simulink model "system_simulation"  (R2024a)
settings: Solver=VariableStepAuto  StartTime=0.0  StopTime=1  RelTol=1e-3
undefined symbols (not defined in the file or in its folder): A, B, C, F, FI
settings Model: Creator=balder  LastModifiedBy=balder

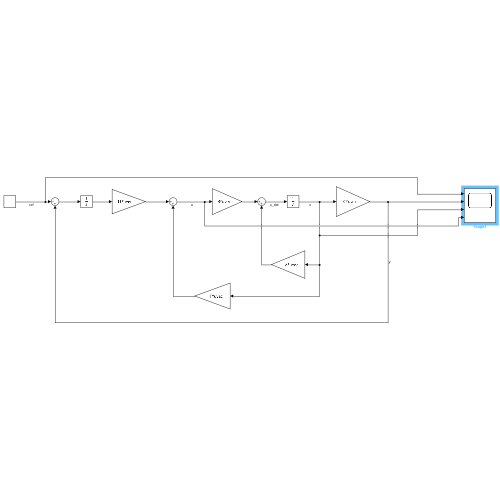
[thumbnail: Simulink's stored preview of the top-level diagram]
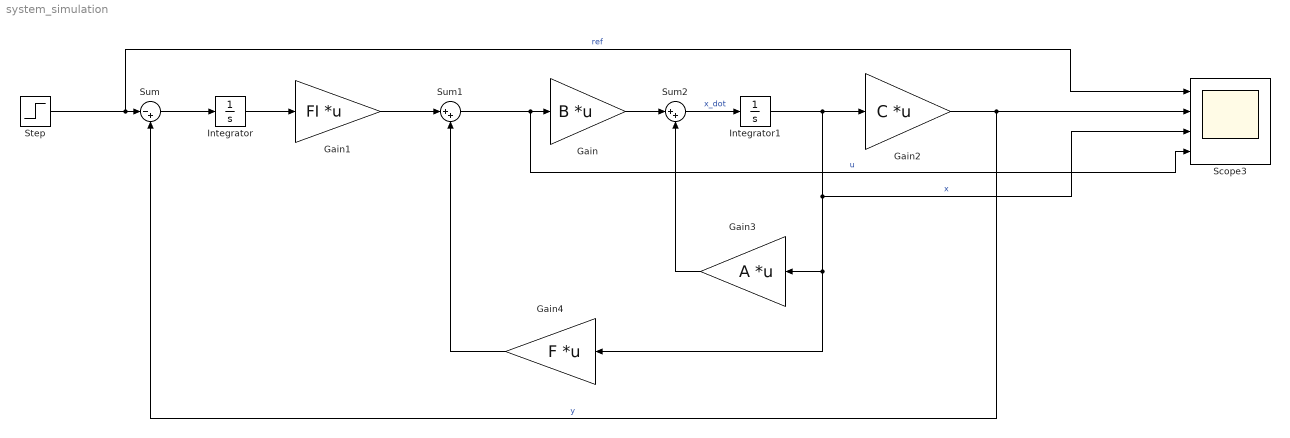
== system system_simulation ==
  Gain : Gain  Gain=B  Multiplication=Matrix(K*u) (u vector)
  Gain1 : Gain  Gain=FI  Multiplication=Matrix(K*u) (u vector)
  Gain2 : Gain  Gain=C  Multiplication=Matrix(K*u) (u vector)
  Gain3 : Gain  Gain=A  Multiplication=Matrix(K*u) (u vector)
  Gain4 : Gain  Gain=F  Multiplication=Matrix(K*u) (u vector)
  Integrator : Integrator
  Integrator1 : Integrator
  Scope3 : Scope  NumInputPorts=4
  Step : Step  Time=0.5  Before=[0 0]  After=[1 -1]  SampleTime=0
  Sum : Sum  Inputs=|-+
  Sum1 : Sum  Inputs=|++
  Sum2 : Sum  Inputs=|++
  wires:
  Sum2/1 -> Integrator1/1  "x_dot"
  Gain/1 -> Sum2/1
  Gain1/1 -> Sum1/1
  Integrator/1 -> Gain1/1
  Sum/1 -> Integrator/1
  Gain3/1 -> Sum2/2
  Step/1 -> Scope3/1, Sum/1  "ref"
  Sum1/1 -> Scope3/4, Gain/1  "u"
  Gain2/1 -> Scope3/2, Sum/2  "y"
  Gain4/1 -> Sum1/2
  Integrator1/1 -> Scope3/3, Gain4/1, Gain3/1, Gain2/1  "x"
